simulink model "Frame_transformation_s"  (R2024b)
settings: Solver=VariableStepAuto  StartTime=0.0  StopTime=64  RelTol=1e-3
values from neighbouring files (symbols this model uses):
  C = [1 0 0 0; 0 1 0 0]    [Car_test_UDP.m]    (also in Final_Code_GPS.m; Final_Code_plotting_reset_kalman.m; KalmanFilter.m)
libraries: sim3dautolib x2, sim3dlib x1
settings Model: Creator=ritvi  LastModifiedBy=ritvi

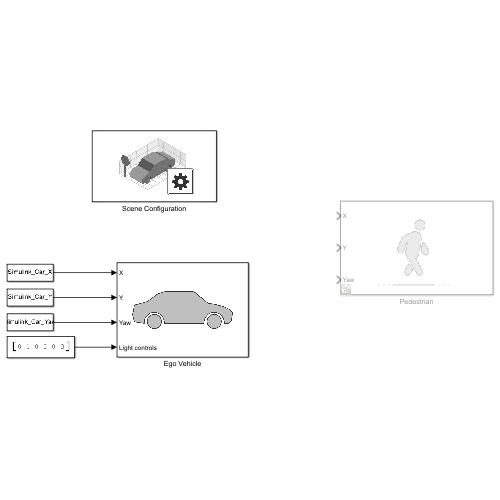
[thumbnail: Simulink's stored preview of the top-level diagram]
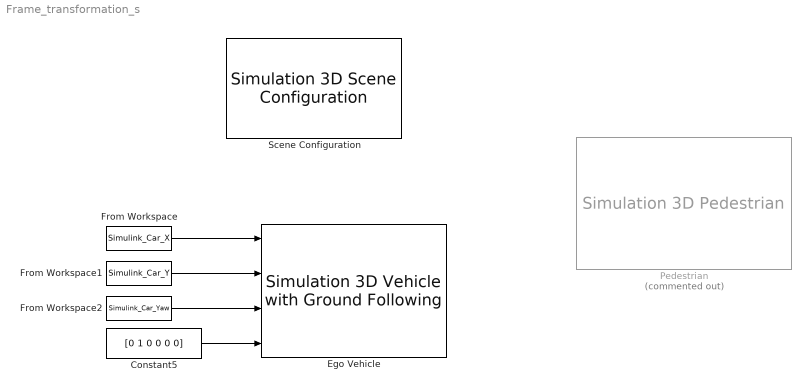
== system Frame_transformation_s ==
  Constant5 : Constant  Value=[0 1 0 0 0 0]
  Ego Vehicle : sim3dautolib/Simulation 3D Vehicle with Ground Following  Priority=-1  PassVehMesh=Hatchback  MeshPath=/MathWorksSimulation/Vehicles/Muscle/Meshes/SK_MuscleCar.SK_MuscleCar  TrackWidth=1.9  WheelBase=3  WheelRadius=0.35  VehColor=Red  InitialPos=[50, 50, 0]  InitialRot=[0, 0, 90]  ActorName=SimulinkVehicle1  SampleTime=-1  ActorType=SimulinkVehicle  ID=1  aMode=3  ActorTag=SimulinkVehicle1  CoordinateScheme=ISO  VehLightsControl=on  HeadlightColor=[ 1, 1, 1 ]  HighBeamIntensity=100000  LowBeamIntensity=60000  HighBeamConeAngle=70  LowBeamConeAngle=70  LeftHeadlightOrientation=[ 0, 0 ]  RightHeadlightOrientation=[ 0, 0 ]  BrakelightIntensity=500  ReverselightIntensity=500  SignallightIntensity=500  SignallightPeriod=1  SignalPulseWidth=50  TransformOutportEnabled=off
      settings: LibrarySourceBlock=drivingsim3d/Simulation 3D Vehicle with Ground Following
  From Workspace : FromWorkspace  VariableName=Simulink_Car_X
  From Workspace1 : FromWorkspace  VariableName=Simulink_Car_Y
  From Workspace2 : FromWorkspace  VariableName=Simulink_Car_Yaw
  Pedestrian : sim3dautolib/Simulation 3D Pedestrian  Priority=-1  Commented=on  PedestrianType=Female 1  Scale=[1, 1, 1]  InitialPos=[0, 0, 0]  InitialYaw=0  ActorName=SimulinkPedestrian1  SampleTime=-1  ActorType=SimulinkPedestrian  ActorTag=SimulinkPedestrian1  ID=1  aMode=3  CoordinateScheme=ISO  TransformOutportEnabled=off
      settings: LibrarySourceBlock=drivingsim3d/Simulation 3D Pedestrian
  Scene Configuration : sim3dlib/Simulation 3D Scene Configuration  Priority=0  ProjectFormat=Unreal Editor  SceneDesc=Large parking lot  ProjectName=C:\Program Files\MATLAB\R2024b\toolbox\shared\sim3d_projects\automotive_project_windows\UE\WindowsNoEditor\VehicleSimulation.exe  ScenePath=/Game/Maps/HwStrght  UEProjPath=C:\Local\AutoVrtlEnv\AutoVrtlEnv.uproject  EnableOpenDRIVE=off  vehTagList={'Custom';'Scene Origin';'SimulinkVehicle1'}  vehTag=SimulinkVehicle1  FreeCameraInitialTranslation=[0, 0, 0]  FreeCameraDefaultInitialTranslation=[-6, 0, 2]  FreeCameraInitialRotation=[0, 0, 0]  FreeCameraDefaultInitialRotation=[0, -15, 0]  OpVisEn=off  Ts=0.05  EnableWindow=on  EnableRemoteAccess=off  EnableWeather=off  SunAzimuth=183.600  SunAltitude=0.0  EnableGeospatialSun=off  Latitude=0  Longitude=0  Date=2023-01-01  Time=10:30:00  GeoTimeZone=-5.0  SunDaylightSaving=off  wind=1  clouds=50.0  EnableVolumetricClouds=off  CloudCoverage=0  CloudAltitude=6  fog=0.0  rain=18.0  RaindropsEffect=off  SnowDensity=0  EnableGeospatial=off  UseTrueOrigin=off  OriginHeight=200  OriginLatitude=40.744652  OriginLongitude=-73.988864  MapStyle=Aerial  AdditionalAssetIDs=[]  UseAdvancedSunSky=off  SolarTime=11  TimeZone=-5  Day=21  Month=9  Year=2022  UseDaylightSavingTime=on  DSTStartDay=10  DSTStartMonth=3  DSTEndDay=3  DSTEndMonth=11  DSTSwitchHour=2  sensorTag=MainCamera1  sensorId=1  sensorName=MainCamera1  mountLoc=Origin  offsetFlag=off  tmountOffset=[0, 0, 0]  rmountOffset=[0, 0, 0]  HorizontalResolution=1280  VerticalResolution=720  HorizontalFOV=60  mountPoint=[0 0 0]  mountOrientation=[0 0 0]  aMode=3  ID=1  GeoTrigger=Inactive
      settings: LibrarySourceBlock=drivingsim3d/Simulation 3D Scene Configuration
  wires:
  Constant5/1 -> Ego Vehicle/4
  From Workspace2/1 -> Ego Vehicle/3
  From Workspace/1 -> Ego Vehicle/1
  From Workspace1/1 -> Ego Vehicle/2
